simulink library "SCA_SimulinkHIL_lib"  (R2023b)
settings: Solver=VariableStepAuto  StartTime=0.0  StopTime=10.0  RelTol=1e-3
undefined symbols (not defined in the file): a, b, c, DiscIntNeverNeededParam, n
libraries: simulink x11, hdlsllib x8, $bdroot x6, fpga_utils_lib x4
settings Model: Creator=promero  LastModifiedBy=promero

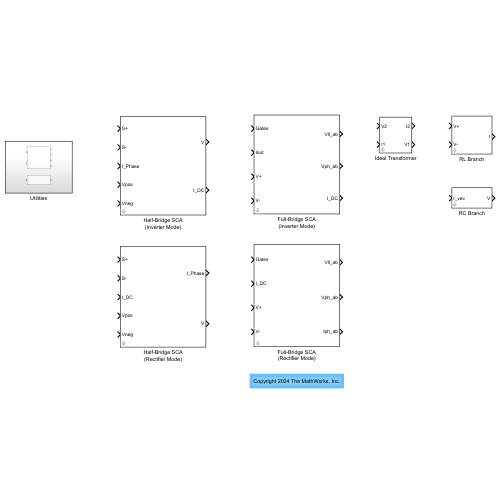
[thumbnail: Simulink's stored preview of the top-level diagram]
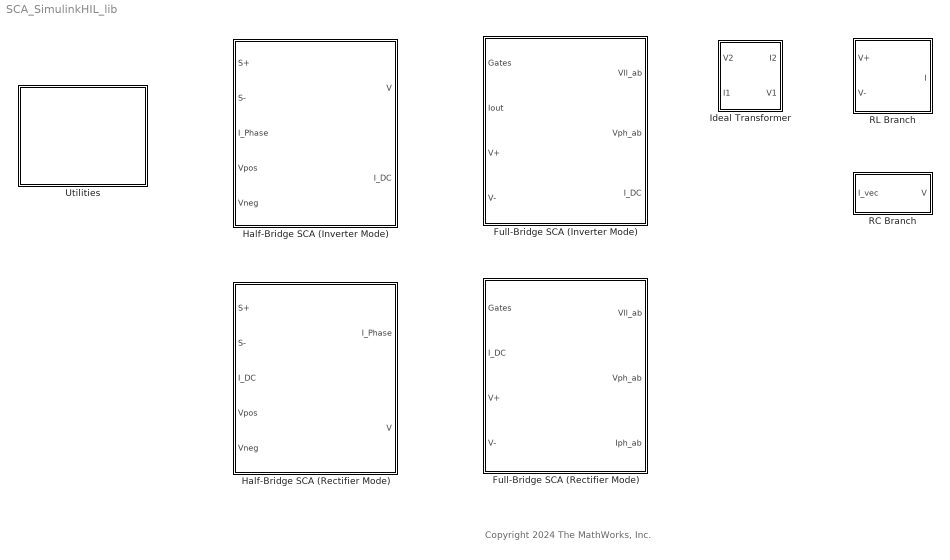
== system SCA_SimulinkHIL_lib ==
  note: Copyright 2024 The MathWorks, Inc.
  Full-Bridge SCA (Inverter Mode) : Subsystem  mask{vfSwitch=0.5, rSwitch=0.001, vfDiode=0.8, rDiode=0.001, avgRatio=1, rSnub=100, useFixedP=on}
      mask prompts: vfSwitch "Switch Threshold [V]"; rSwitch "Switch Closed Resistance [Ohms]"; vfDiode "Diode Forward Voltage [V]"; rDiode "Diode On Resistance [Ohms]"; avgRatio "Subcycle Average Factor [-]"; rSnub "Snubber Resistance [Ohms]"; useFixedP "Use fixed-point implementation"
      mask TypeOptions vfSwitch: Half-Bridge SCA Phase A/vfSwitch | Half-Bridge SCA Phase B/vfSwitch
      mask TypeOptions rSwitch: Half-Bridge SCA Phase A/rSwitch | Half-Bridge SCA Phase B/rSwitch
      mask TypeOptions vfDiode: Half-Bridge SCA Phase A/vfDiode | Half-Bridge SCA Phase B/vfDiode
      mask TypeOptions rDiode: Half-Bridge SCA Phase A/rDiode | Half-Bridge SCA Phase B/rDiode
      mask TypeOptions avgRatio: Half-Bridge SCA Phase A/avgRatio | Half-Bridge SCA Phase B/avgRatio
      mask TypeOptions rSnub: Half-Bridge SCA Phase A/rSnub | Half-Bridge SCA Phase B/rSnub
      mask TypeOptions useFixedP: Half-Bridge SCA Phase A/useFixedP | Half-Bridge SCA Phase B/useFixedP
      mask DialogControl ParameterGroupVar Prompt: Physical Paramaters
      mask DialogControl Container3 Prompt: Simulation Parameters
  Full-Bridge SCA (Rectifier Mode) : Subsystem  mask{vfSwitch=0.5, rSwitch=0.001, cSwitch=1e-8, vfDiode=0.6, rDiode=0.3, cDiode=1e-8, avgRatio=1, rSnubber=1000, useFixedP=on}
      mask prompts: vfSwitch "Switch Threshold [V]"; rSwitch "Switch Closed Resistance [Ohm]"; cSwitch "Switch Open Conductance [1/Ohm]"; vfDiode "Diode Forward Voltage [V]"; rDiode "Diode On Resistance [Ohm]"; cDiode "Diode Off Conductance [1/Ohm]"; avgRatio "Window length"; rSnubber "Snubber Resistance [Ohm]"; useFixedP "Use fixed-point implementation"
      mask TypeOptions vfSwitch:
      | Half-Bridge SCA Phase A
      | (Rectifier Mode)/vfSwitch | Half-Bridge SCA Phase B
      | (Rectifier Mode)/vfSwitch
      mask TypeOptions rSwitch:
      | Half-Bridge SCA Phase A
      | (Rectifier Mode)/rSwitch | Half-Bridge SCA Phase B
      | (Rectifier Mode)/rSwitch
      mask TypeOptions cSwitch:
      | Half-Bridge SCA Phase A
      | (Rectifier Mode)/cSwitch | Half-Bridge SCA Phase B
      | (Rectifier Mode)/cSwitch
      mask TypeOptions vfDiode:
      | Half-Bridge SCA Phase A
      | (Rectifier Mode)/vfDiode | Half-Bridge SCA Phase B
      | (Rectifier Mode)/vfDiode
      mask TypeOptions rDiode:
      | Half-Bridge SCA Phase A
      | (Rectifier Mode)/rDiode | Half-Bridge SCA Phase B
      | (Rectifier Mode)/rDiode
      mask TypeOptions cDiode:
      | Half-Bridge SCA Phase A
      | (Rectifier Mode)/cDiode | Half-Bridge SCA Phase B
      | (Rectifier Mode)/cDiode
      mask TypeOptions avgRatio:
      | Half-Bridge SCA Phase A
      | (Rectifier Mode)/avgRatio | Half-Bridge SCA Phase B
      | (Rectifier Mode)/avgRatio
      mask TypeOptions rSnubber:
      | Half-Bridge SCA Phase A
      | (Rectifier Mode)/rSnubber | Half-Bridge SCA Phase B
      | (Rectifier Mode)/rSnubber
      mask TypeOptions useFixedP:
      | Half-Bridge SCA Phase A
      | (Rectifier Mode)/useFixedP | Half-Bridge SCA Phase B
      | (Rectifier Mode)/useFixedP
      mask DialogControl ParameterGroupVar Prompt: Physical Paramaters
      mask DialogControl Container3 Prompt: Simulation Parameters
  Half-Bridge SCA (Inverter Mode) : Subsystem  mask{vfSwitch=0.5, rSwitch=0.001, vfDiode=0.8, rDiode=0.001, avgRatio=1, useFixedP=on, rSnub=100}
      mask prompts: vfSwitch "Switch Threshold [V]"; rSwitch "Switch Closed Resistance [Ohm]"; vfDiode "Diode Forward Voltage [V]"; rDiode "Diode On Resistance [Ohm]"; avgRatio "Window length"; useFixedP "Use fixed-point implementation"; rSnub "Snubber Resistance [Ohm]"
      mask init:
      | if useFixedP
      |     set_param([gcb,'/Data Type Conversion'],"Commented","through");
      |     set_param([gcb,'/Data Type Conversion1'],"Commented","through");
      |     set_param([gcb,'/Data Type Conversion2'],"Commented","through");
      | else
      |     set_param([gcb,'/Data Type Conversion'],"Commented","off");
      |     set_param([gcb,'/Data Type Conversion1'],"Commented","off");
      |     set_param([gcb,'/Data Type Conversion2'],"Commented","off");
      | end
      mask TypeOptions avgRatio: Switch State Average/avgRatio
      mask DialogControl ParameterGroupVar Prompt: Physical Parameters
      mask DialogControl Container3 Prompt: Simulation Parameters
  Half-Bridge SCA (Rectifier Mode) : Subsystem  mask{vfSwitch=0.5, rSwitch=0.001, cSwitch=1e-8, vfDiode=0.6, rDiode=0.3, cDiode=1e-8, avgRatio=1, useFixedP=on, rSnubber=inf}
      mask prompts: vfSwitch "Switch Threshold [V]"; rSwitch "Switch Closed Resistance [Ohm]"; cSwitch "Switch Open Conductance [1/Ohm]"; vfDiode "Diode Forward Voltage [V]"; rDiode "Diode On Resistance [Ohm]"; cDiode "Diode Off Conductance [1/Ohm]"; avgRatio "Window length"; useFixedP "Use fixed-point implementation"; rSnubber "Snubber Resistance [Ohm]"
      mask init:
      | if rDiode > 0
      |     rEquiv = 1/(1/rSwitch + 1/rDiode);
      | else
      |     rEquiv = rSwitch;
      | end
      | 
      | if useFixedP
      |     set_param([gcb,'/Data Type Conversion'],"Commented","through");
      |     set_param([gcb,'/Data Type Conversion1'],"Commented","through");
      |     set_param([gcb,'/Data Type Conversion2'],"Commented","through");
      | else
      |     set_param([gcb,'/Data Type Conversion'],"Commented","off");
      |     set_param([gcb,'/Data Type Conversion1'],"Commented","off");
      |     set_param([gcb,'/Data Type Conversion2'],"Commented","off");
      | end
      mask TypeOptions avgRatio: Switch State Average/avgRatio
      mask DialogControl ParameterGroupVar Prompt: Physical Parameters
      mask DialogControl Container3 Prompt: Simulation Parameters
  Ideal Transformer : Subsystem  mask(Ideal Transformer){Parameter1=1}
      mask prompts: Parameter1 "Winding ratio [-]"
  RC Branch : Subsystem  mask(RC Branch){C=1e-4, R=0.1}
      mask prompts: C "Capacitance [F]"; R "Resistance [Ohm]"
  RL Branch : Subsystem  mask(RL Branch){L=1e-6, R=0}
      mask prompts: L "Inductance [H]"; R "Resistance [Ohm]"
  Utilities : Subsystem

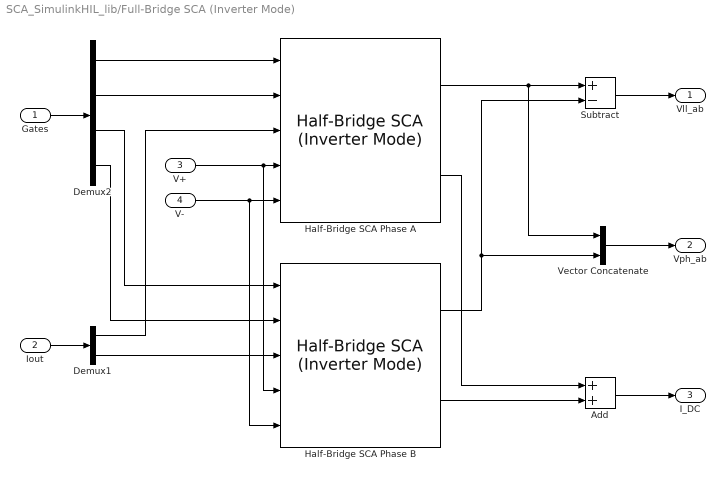
== system SCA_SimulinkHIL_lib/Full-Bridge SCA (Inverter Mode) ==
  Gates : Inport  OutDataTypeStr=boolean  PortDimensions=4
  Iout : Inport  Port=2  PortDimensions=2
  V+ : Inport  Port=3  PortDimensions=1
  V- : Inport  Port=4  PortDimensions=1
  Add : Sum
  Demux1 : Demux  Outputs=2
  Demux2 : Demux
  Half-Bridge SCA Phase A : $bdroot/Half-Bridge SCA (Inverter Mode)  vfSwitch=vfSwitch  rSwitch=rSwitch  vfDiode=vfDiode  rDiode=rDiode  avgRatio=avgRatio  useFixedP=on  rSnub=rSnub
  Half-Bridge SCA Phase B : $bdroot/Half-Bridge SCA (Inverter Mode)  vfSwitch=vfSwitch  rSwitch=rSwitch  vfDiode=vfDiode  rDiode=rDiode  avgRatio=avgRatio  useFixedP=on  rSnub=rSnub
  Subtract : Sum  Inputs=+-
  Vector Concatenate : Concatenate
  Vll_ab : Outport
  Vph_ab : Outport  Port=2
  I_DC : Outport  Port=3
  wires:
  Demux2/2 -> Half-Bridge SCA Phase A/2
  Demux2/1 -> Half-Bridge SCA Phase A/1
  Gates/1 -> Demux2/1
  Demux2/3 -> Half-Bridge SCA Phase B/1
  Demux2/4 -> Half-Bridge SCA Phase B/2
  Iout/1 -> Demux1/1
  Demux1/1 -> Half-Bridge SCA Phase A/3
  Demux1/2 -> Half-Bridge SCA Phase B/3
  V+/1 -> Half-Bridge SCA Phase B/4, Half-Bridge SCA Phase A/4
  V-/1 -> Half-Bridge SCA Phase B/5, Half-Bridge SCA Phase A/5
  Half-Bridge SCA Phase A/2 -> Add/1
  Half-Bridge SCA Phase B/2 -> Add/2
  Add/1 -> I_DC/1
  Half-Bridge SCA Phase A/1 -> Vector Concatenate/1, Subtract/1
  Half-Bridge SCA Phase B/1 -> Vector Concatenate/2, Subtract/2
  Subtract/1 -> Vll_ab/1
  Vector Concatenate/1 -> Vph_ab/1

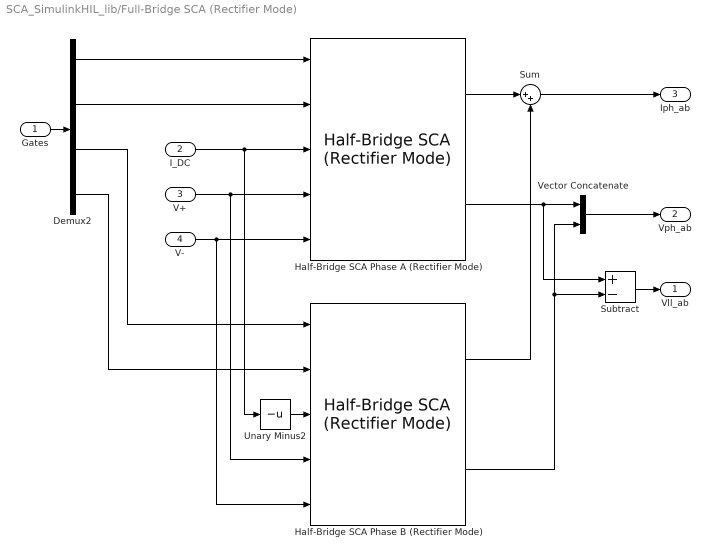
== system SCA_SimulinkHIL_lib/Full-Bridge SCA (Rectifier Mode) ==
  Gates : Inport  PortDimensions=4
  I_DC : Inport  Port=2  PortDimensions=1
  V+ : Inport  Port=3  PortDimensions=1
  V- : Inport  Port=4  PortDimensions=1
  Demux2 : Demux
  Half-Bridge SCA Phase A (Rectifier Mode) : $bdroot/Half-Bridge SCA (Rectifier Mode)  vfSwitch=vfSwitch  rSwitch=rSwitch  cSwitch=cSwitch  vfDiode=vfDiode  rDiode=rDiode  cDiode=cDiode  avgRatio=avgRatio  useFixedP=on  rSnubber=rSnubber
  Half-Bridge SCA Phase B (Rectifier Mode) : $bdroot/Half-Bridge SCA (Rectifier Mode)  vfSwitch=vfSwitch  rSwitch=rSwitch  cSwitch=cSwitch  vfDiode=vfDiode  rDiode=rDiode  cDiode=cDiode  avgRatio=avgRatio  useFixedP=on  rSnubber=rSnubber
  Subtract : Sum  Inputs=+-  OutDataTypeStr=Inherit: Inherit via back propagation
  Sum : Sum  Inputs=|++
  Unary Minus2 : UnaryMinus
  Vector Concatenate : Concatenate
  Vll_ab : Outport
  Vph_ab : Outport  Port=2
  Iph_ab : Outport  Port=3
  wires:
  V-/1 -> Half-Bridge SCA Phase A (Rectifier Mode)/5, Half-Bridge SCA Phase B (Rectifier Mode)/5
  V+/1 -> Half-Bridge SCA Phase A (Rectifier Mode)/4, Half-Bridge SCA Phase B (Rectifier Mode)/4
  I_DC/1 -> Half-Bridge SCA Phase A (Rectifier Mode)/3, Unary Minus2/1
  Unary Minus2/1 -> Half-Bridge SCA Phase B (Rectifier Mode)/3
  Half-Bridge SCA Phase B (Rectifier Mode)/2 -> Subtract/2, Vector Concatenate/2
  Vector Concatenate/1 -> Vph_ab/1
  Sum/1 -> Iph_ab/1
  Half-Bridge SCA Phase A (Rectifier Mode)/2 -> Subtract/1, Vector Concatenate/1
  Half-Bridge SCA Phase B (Rectifier Mode)/1 -> Sum/2
  Half-Bridge SCA Phase A (Rectifier Mode)/1 -> Sum/1
  Demux2/4 -> Half-Bridge SCA Phase B (Rectifier Mode)/2
  Gates/1 -> Demux2/1
  Demux2/2 -> Half-Bridge SCA Phase A (Rectifier Mode)/2
  Demux2/1 -> Half-Bridge SCA Phase A (Rectifier Mode)/1
  Demux2/3 -> Half-Bridge SCA Phase B (Rectifier Mode)/1
  Subtract/1 -> Vll_ab/1

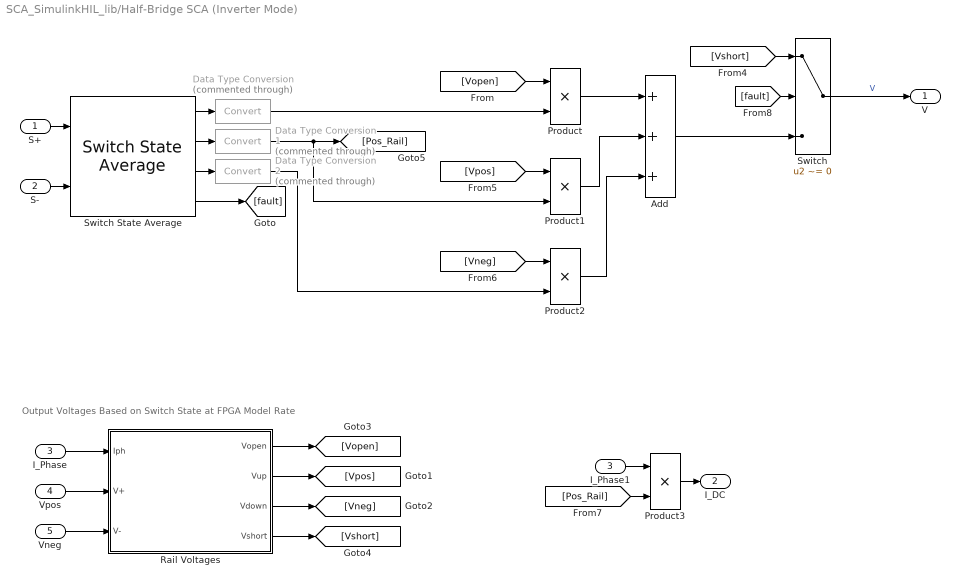
== system SCA_SimulinkHIL_lib/Half-Bridge SCA (Inverter Mode) ==
  note: Output Voltages Based on Switch State at FPGA Model Rate
  S+ : Inport
  S- : Inport  Port=2
  I_Phase : Inport  Port=3
  Vpos : Inport  Port=4
  Vneg : Inport  Port=5
  Add : Sum  Inputs=+++  OutDataTypeStr=Inherit: Inherit via back propagation
  Data Type Conversion : DataTypeConversion  Commented=through  SaturateOnIntegerOverflow=off  RndMeth=Floor
  Data Type Conversion1 : DataTypeConversion  Commented=through  SaturateOnIntegerOverflow=off  RndMeth=Floor
  Data Type Conversion2 : DataTypeConversion  Commented=through  SaturateOnIntegerOverflow=off  RndMeth=Floor
  I_Phase1 : InportShadow  Port=3
  Product{,1..3} (4 alike) : Product  OutDataTypeStr=Inherit: Same as first input
  Rail Voltages : Subsystem
  Switch : Switch  Criteria=u2 ~= 0  SaturateOnIntegerOverflow=off
  Switch State Average : $bdroot/Utilities/Switch State Average  avgRatio=avgRatio
  V : Outport  VectorParamsAs1DForOutWhenUnconnected=off
  I_DC : Outport  Port=2  VectorParamsAs1DForOutWhenUnconnected=off
  wires:
  [Vshort] -> Switch/1
  Switch/1 -> V/1  "V"
  [fault] -> Switch/2
  Switch State Average/2 -> Data Type Conversion1/1
  [Vpos] -> Product1/1
  [Pos_Rail] -> Product3/2
  I_Phase1/1 -> Product3/1
  Vpos/1 -> Rail Voltages/2(V+)
  Vneg/1 -> Rail Voltages/3(V-)
  Rail Voltages/1(Vopen) -> [Vopen]
  Rail Voltages/2(Vup) -> [Vpos]
  Rail Voltages/3(Vdown) -> [Vneg]
  Rail Voltages/4(Vshort) -> [Vshort]
  Switch State Average/4 -> [fault]
  S+/1 -> Switch State Average/1
  S-/1 -> Switch State Average/2
  Add/1 -> Switch/3
  I_Phase/1 -> Rail Voltages/1(Iph)
  [Vopen] -> Product/1
  Switch State Average/1 -> Data Type Conversion/1
  Product/1 -> Add/1
  [Vneg] -> Product2/1
  Switch State Average/3 -> Data Type Conversion2/1
  Product1/1 -> Add/2
  Product2/1 -> Add/3
  Product3/1 -> I_DC/1
  Data Type Conversion/1 -> Product/2
  Data Type Conversion1/1 -> Product1/2, [Pos_Rail]
  Data Type Conversion2/1 -> Product2/2

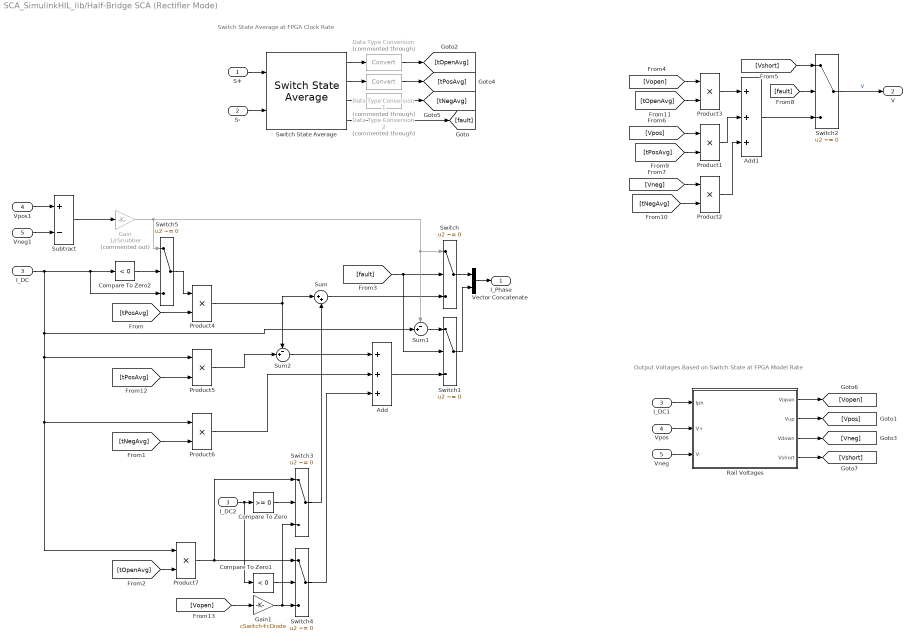
== system SCA_SimulinkHIL_lib/Half-Bridge SCA (Rectifier Mode) ==
  note: Switch State Average at FPGA Clock Rate
  note: Output Voltages Based on Switch State at FPGA Model Rate
  S+ : Inport  PortDimensions=1
  S- : Inport  Port=2  PortDimensions=1
  I_DC : Inport  Port=3
  Vpos : Inport  Port=4
  Vneg : Inport  Port=5
  Add : Sum  Inputs=+++  OutDataTypeStr=Inherit: Inherit via back propagation
  Add1 : Sum  Inputs=+++  OutDataTypeStr=Inherit: Inherit via back propagation  InputSameDT=on
  Compare To Zero : simulink/Logic and Bit Operations/Compare To Zero  relop=>=  OutDataTypeStr=boolean
  Compare To Zero1 : simulink/Logic and Bit Operations/Compare To Zero  relop=<  OutDataTypeStr=boolean
  Compare To Zero2 : simulink/Logic and Bit Operations/Compare To Zero  relop=<  OutDataTypeStr=boolean
  Data Type Conversion : DataTypeConversion  Commented=through  SaturateOnIntegerOverflow=off  RndMeth=Floor
  Data Type Conversion1 : DataTypeConversion  Commented=through  SaturateOnIntegerOverflow=off  RndMeth=Floor
  Data Type Conversion2 : DataTypeConversion  Commented=through  SaturateOnIntegerOverflow=off  RndMeth=Floor
  Gain : Gain  Commented=on  Gain=1/rSnubber  OutDataTypeStr=Inherit: Inherit via back propagation
  Gain1 : Gain  Gain=cSwitch+cDiode  OutDataTypeStr=Inherit: Inherit via back propagation
  I_DC1 : InportShadow  Port=3
  I_DC2 : InportShadow  Port=3
  Product{1..7} (7 alike) : Product  OutDataTypeStr=Inherit: Same as first input
  Rail Voltages : Subsystem
  Subtract : Sum  Inputs=+-
  Sum : Sum  Inputs=|++  OutDataTypeStr=Inherit: Inherit via back propagation
  Sum1 : Sum  Inputs=-+|  OutDataTypeStr=Inherit: Inherit via back propagation
  Sum2 : Sum  Inputs=-+|
  Switch{,1..5} (6 alike) : Switch  Criteria=u2 ~= 0  SaturateOnIntegerOverflow=off
  Switch State Average : $bdroot/Utilities/Switch State Average  avgRatio=avgRatio
  Vector Concatenate : Concatenate
  Vneg1 : InportShadow  Port=5
  Vpos1 : InportShadow  Port=4
  I_Phase : Outport
  V : Outport  Port=2  VectorParamsAs1DForOutWhenUnconnected=off
  wires:
  Sum2/1 -> Add/1
  Switch4/1 -> Add/3
  Add/1 -> Switch1/3
  Switch5/1 -> Product4/1
  Compare To Zero2/1 -> Switch5/2
  Compare To Zero1/1 -> Switch4/2
  Switch3/1 -> Sum/2
  Product7/1 -> Switch3/1, Switch4/1
  Compare To Zero/1 -> Switch3/2
  I_DC2/1 -> Compare To Zero/1, Compare To Zero1/1
  Vneg1/1 -> Subtract/2
  Vpos1/1 -> Subtract/1
  Sum1/1 -> Switch1/1
  [fault] -> Switch1/2, Switch/2
  Sum/1 -> Switch/3
  I_DC/1 -> Compare To Zero2/1, Switch5/3, Product5/1, Product7/1, Product6/1, Sum1/2
  [tPosAvg] -> Product4/2
  Switch State Average/1 -> Data Type Conversion/1
  Switch State Average/2 -> Data Type Conversion1/1
  Switch State Average/3 -> Data Type Conversion2/1
  Switch State Average/4 -> [fault]
  Rail Voltages/4(Vshort) -> [Vshort]
  Vneg/1 -> Rail Voltages/3(V-)
  Vpos/1 -> Rail Voltages/2(V+)
  Rail Voltages/1(Vopen) -> [Vopen]
  Rail Voltages/2(Vup) -> [Vpos]
  I_DC1/1 -> Rail Voltages/1(Iph)
  Rail Voltages/3(Vdown) -> [Vneg]
  [Vopen] -> Product3/1
  Switch2/1 -> V/1  "V"
  Add1/1 -> Switch2/3
  [Vshort] -> Switch2/1
  [Vneg] -> Product2/1
  [fault] -> Switch2/2
  [tOpenAvg] -> Product3/2
  [tNegAvg] -> Product2/2
  Vector Concatenate/1 -> I_Phase/1
  Switch/1 -> Vector Concatenate/1
  Switch1/1 -> Vector Concatenate/2
  S+/1 -> Switch State Average/1
  S-/1 -> Switch State Average/2
  Subtract/1 -> Gain/1
  Gain/1 -> Switch/1, Sum1/1, Switch5/1
  [Vopen] -> Gain1/1
  Gain1/1 -> Switch4/3, Switch3/3
  [Vpos] -> Product1/1
  [tPosAvg] -> Product1/2
  Product3/1 -> Add1/1
  Product1/1 -> Add1/2
  Product2/1 -> Add1/3
  Product4/1 -> Sum/1, Sum2/1
  Product5/1 -> Sum2/2
  [tPosAvg] -> Product5/2
  [tNegAvg] -> Product6/2
  Product6/1 -> Add/2
  [tOpenAvg] -> Product7/2
  Data Type Conversion/1 -> [tOpenAvg]
  Data Type Conversion1/1 -> [tPosAvg]
  Data Type Conversion2/1 -> [tNegAvg]

== system SCA_SimulinkHIL_lib/Ideal Transformer ==
  V2 : Inport  PortDimensions=1
  I1 : Inport  Port=2
  Gain1 : Gain  Gain=n  OutDataTypeStr=Inherit: Inherit via back propagation
  Gain2 : Gain  Gain=n  OutDataTypeStr=Inherit: Inherit via back propagation
  I2 : Outport
  V1 : Outport  Port=2
  wires:
  V2/1 -> Gain2/1
  Gain2/1 -> V1/1
  Gain1/1 -> I2/1
  I1/1 -> Gain1/1

== system SCA_SimulinkHIL_lib/RC Branch ==
  I_vec : Inport
  Constant : Constant  Value=R  OutDataTypeStr=Inherit: Inherit via back propagation  SampleTime=Inf
  Data Type Duplicate : DataTypeDuplicate
  Discrete-Time Integrator : DiscreteIntegrator  gainval=1/C  SampleTime=-1  OutDataTypeStr=Inherit: Inherit via back propagation  ICPrevOutput=DiscIntNeverNeededParam  ICPrevScaledInput=DiscIntNeverNeededParam
  Multiply-Add : hdlsllib/HDL Operations/Multiply-Add  Function=c-(a.*b)  datatype=Inherit: Inherit via back propagation  DoSatur=off  FMA=off
  Sum of Elements : Sum  Inputs=+
  V : Outport
  wires:
  Sum of Elements/1 -> Multiply-Add/1, Discrete-Time Integrator/1
  I_vec/1 -> Sum of Elements/1
  Constant/1 -> Multiply-Add/2
  Discrete-Time Integrator/1 -> Data Type Duplicate/2, Multiply-Add/3
  Multiply-Add/1 -> Data Type Duplicate/1, V/1

== system SCA_SimulinkHIL_lib/RL Branch ==
  V+ : Inport  PortDimensions=1
  V- : Inport  Port=2  PortDimensions=1
  Discrete-Time Integrator : DiscreteIntegrator  gainval=1/L  SampleTime=-1  OutDataTypeStr=Inherit: Inherit via back propagation  ICPrevOutput=DiscIntNeverNeededParam  ICPrevScaledInput=DiscIntNeverNeededParam
  Gain : Gain  Gain=R  OutDataTypeStr=Inherit: Inherit via back propagation
  Subtract : Sum  Inputs=+--  OutDataTypeStr=Inherit: Inherit via back propagation
  Unit Delay : UnitDelay  SampleTime=-1  HasFrameUpgradeWarning=on
  I : Outport
  wires:
  Discrete-Time Integrator/1 -> Gain/1, I/1
  V+/1 -> Subtract/1
  Subtract/1 -> Discrete-Time Integrator/1
  V-/1 -> Subtract/2
  Gain/1 -> Unit Delay/1
  Unit Delay/1 -> Subtract/3

== system SCA_SimulinkHIL_lib/Utilities ==
  Fast to Slow Transition : Subsystem  mask{avgRatio=1}
      mask prompts: avgRatio "Time scaling factor"
      mask TypeOptions avgRatio: HDL Moving Average/avgRatio | Rate Transition/OutPortSampleTimeMultiple
  Switch State Average : Subsystem  mask{avgRatio=1}
      mask prompts: avgRatio "Window length"
      mask TypeOptions avgRatio: Subsystem/Moving Average/HDL Moving Average/avgRatio | Subsystem/Moving Average/HDL Moving Average1/avgRatio | Subsystem/Moving Average/HDL Moving Average2/avgRatio
      mask DialogControl Container3 Prompt: Parameters

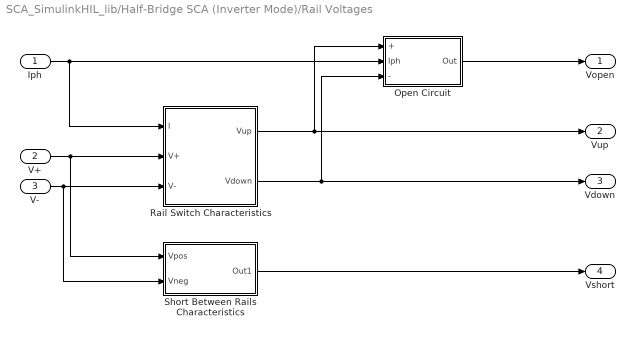
== system SCA_SimulinkHIL_lib/Half-Bridge SCA (Inverter Mode)/Rail Voltages ==
  Iph : Inport
  V+ : Inport  Port=2
  V- : Inport  Port=3
  Open Circuit : Subsystem
  Rail Switch Characteristics : Subsystem
  Short Between Rails Characteristics : Subsystem
  Vopen : Outport
  Vup : Outport  Port=2
  Vdown : Outport  Port=3
  Vshort : Outport  Port=4
  wires:
  Open Circuit/1(Out) -> Vopen/1
  V-/1 -> Short Between Rails Characteristics/2(Vneg), Rail Switch Characteristics/3(V-)
  Rail Switch Characteristics/2(Vdown) -> Open Circuit/3(-), Vdown/1
  Rail Switch Characteristics/1(Vup) -> Open Circuit/1(+), Vup/1
  V+/1 -> Rail Switch Characteristics/2(V+), Short Between Rails Characteristics/1(Vpos)
  Short Between Rails Characteristics/1(Out1) -> Vshort/1
  Iph/1 -> Rail Switch Characteristics/1(I), Open Circuit/2(Iph)

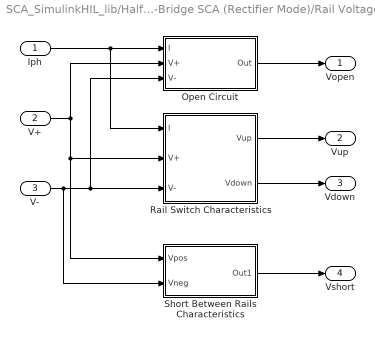
== system SCA_SimulinkHIL_lib/Half-Bridge SCA (Rectifier Mode)/Rail Voltages ==
  Iph : Inport
  V+ : Inport  Port=2
  V- : Inport  Port=3
  Open Circuit : Subsystem
  Rail Switch Characteristics : Subsystem
  Short Between Rails Characteristics : Subsystem
  Vopen : Outport
  Vup : Outport  Port=2
  Vdown : Outport  Port=3
  Vshort : Outport  Port=4
  wires:
  Open Circuit/1(Out) -> Vopen/1
  V-/1 -> Open Circuit/3(V-), Rail Switch Characteristics/3(V-), Short Between Rails Characteristics/2(Vneg)
  Iph/1 -> Rail Switch Characteristics/1(I), Open Circuit/1(I)
  Rail Switch Characteristics/1(Vup) -> Vup/1
  V+/1 -> Short Between Rails Characteristics/1(Vpos), Rail Switch Characteristics/2(V+), Open Circuit/2(V+)
  Short Between Rails Characteristics/1(Out1) -> Vshort/1
  Rail Switch Characteristics/2(Vdown) -> Vdown/1

== system SCA_SimulinkHIL_lib/Utilities/Fast to Slow Transition ==
  In : Inport
  Data Type Duplicate1 : DataTypeDuplicate
  HDL Moving Average : fpga_utils_lib/HDL Moving Average  avgRatio=avgRatio
  Rate Transition : RateTransition  OutPortSampleTimeOpt=Multiple of input port sample time  OutPortSampleTimeMultiple=avgRatio
  Out : Outport
  wires:
  HDL Moving Average/1 -> Data Type Duplicate1/1, Rate Transition/1
  In/1 -> Data Type Duplicate1/2, HDL Moving Average/1
  Rate Transition/1 -> Out/1

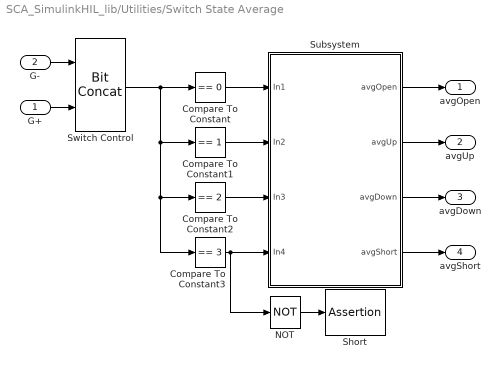
== system SCA_SimulinkHIL_lib/Utilities/Switch State Average ==
  G+ : Inport  OutDataTypeStr=boolean  PortDimensions=1
  G- : Inport  Port=2  OutDataTypeStr=boolean  PortDimensions=1
  Compare To Constant : simulink/Logic and Bit Operations/Compare To Constant  relop===  const=0  OutDataTypeStr=boolean
  Compare To Constant1 : simulink/Logic and Bit Operations/Compare To Constant  relop===  const=1  OutDataTypeStr=boolean
  Compare To Constant2 : simulink/Logic and Bit Operations/Compare To Constant  relop===  const=2  OutDataTypeStr=boolean
  Compare To Constant3 : simulink/Logic and Bit Operations/Compare To Constant  relop===  const=3  OutDataTypeStr=boolean
  NOT : Logic  Operator=NOT  IconShape=distinctive  AllPortsSameDT=off  OutDataTypeStr=boolean
  Short : Assertion  StopWhenAssertionFail=off
  Subsystem : Subsystem  Variant=on  VariantControl=Subsystem
  Switch Control : hdlsllib/Logic and Bit Operations/Bit Concat  numInputs=2
  avgOpen : Outport
  avgUp : Outport  Port=2
  avgDown : Outport  Port=3
  avgShort : Outport  Port=4
  wires:
  Switch Control/1 -> Compare To Constant/1, Compare To Constant3/1, Compare To Constant2/1, Compare To Constant1/1
  NOT/1 -> Short/1
  Compare To Constant3/1 -> NOT/1, Subsystem/4(In4)
  G+/1 -> Switch Control/2
  G-/1 -> Switch Control/1
  Compare To Constant/1 -> Subsystem/1(In1)
  Compare To Constant1/1 -> Subsystem/2(In2)
  Compare To Constant2/1 -> Subsystem/3(In3)
  Subsystem/1(avgOpen) -> avgOpen/1
  Subsystem/2(avgUp) -> avgUp/1
  Subsystem/3(avgDown) -> avgDown/1
  Subsystem/4(avgShort) -> avgShort/1

== system SCA_SimulinkHIL_lib/Half-Bridge SCA (Inverter Mode)/Rail Voltages/Open Circuit ==
  + : Inport
  Iph : Inport  Port=2
  - : Inport  Port=3
  Gain : Gain  Gain=-rSnub
  Saturation Dynamic : simulink/Discontinuities/Saturation Dynamic  OutMin=[]  OutMax=[]  OutDataTypeStr=Inherit: Inherit via back propagation  OutDataType=fixdt(1, 16)  OutScaling=2^-10  DoSatur=off
  Out : Outport  VectorParamsAs1DForOutWhenUnconnected=off
  wires:
  Iph/1 -> Gain/1
  Gain/1 -> Saturation Dynamic/2
  Saturation Dynamic/1 -> Out/1
  +/1 -> Saturation Dynamic/1
  -/1 -> Saturation Dynamic/3

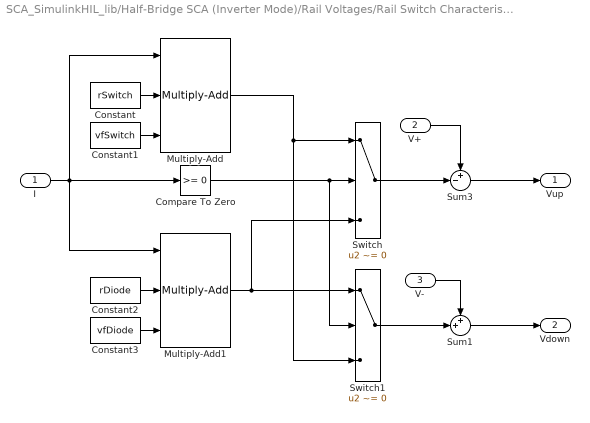
== system SCA_SimulinkHIL_lib/Half-Bridge SCA (Inverter Mode)/Rail Voltages/Rail Switch Characteristics ==
  I : Inport
  V+ : Inport  Port=2
  V- : Inport  Port=3
  Compare To Zero : simulink/Logic and Bit Operations/Compare To Zero  relop=>=  OutDataTypeStr=boolean
  Constant : Constant  Value=rSwitch  OutDataTypeStr=Inherit: Inherit via back propagation
  Constant1 : Constant  Value=vfSwitch  OutDataTypeStr=Inherit: Inherit via back propagation
  Constant2 : Constant  Value=rDiode  OutDataTypeStr=Inherit: Inherit via back propagation
  Constant3 : Constant  Value=vfDiode  OutDataTypeStr=Inherit: Inherit via back propagation
  Multiply-Add : hdlsllib/HDL Operations/Multiply-Add  Function=c+(a.*b)  datatype=Inherit: Inherit via back propagation  DoSatur=off  FMA=off
  Multiply-Add1 : hdlsllib/HDL Operations/Multiply-Add  Function=(a.*b)-c  datatype=Inherit: Inherit via back propagation  DoSatur=off  FMA=off
  Sum1 : Sum  Inputs=++|  OutDataTypeStr=Inherit: Same as first input
  Sum3 : Sum  Inputs=+-|  OutDataTypeStr=Inherit: Same as first input
  Switch : Switch  Criteria=u2 ~= 0  SaturateOnIntegerOverflow=off  InputSameDT=off
  Switch1 : Switch  Criteria=u2 ~= 0  SaturateOnIntegerOverflow=off  InputSameDT=off
  Vup : Outport  VectorParamsAs1DForOutWhenUnconnected=off
  Vdown : Outport  Port=2  VectorParamsAs1DForOutWhenUnconnected=off
  wires:
  Switch/1 -> Sum3/2
  V+/1 -> Sum3/1
  Sum3/1 -> Vup/1
  I/1 -> Compare To Zero/1, Multiply-Add/1, Multiply-Add1/1
  Switch1/1 -> Sum1/2
  Sum1/1 -> Vdown/1
  V-/1 -> Sum1/1
  Compare To Zero/1 -> Switch1/2, Switch/2
  Multiply-Add/1 -> Switch1/3, Switch/1
  Constant/1 -> Multiply-Add/2
  Constant1/1 -> Multiply-Add/3
  Multiply-Add1/1 -> Switch/3, Switch1/1
  Constant2/1 -> Multiply-Add1/2
  Constant3/1 -> Multiply-Add1/3

== system SCA_SimulinkHIL_lib/Half-Bridge SCA (Inverter Mode)/Rail Voltages/Short Between Rails Characteristics ==
  Vpos : Inport
  Vneg : Inport  Port=2
  Gain : Gain  Gain=1/2  OutDataTypeStr=Inherit: Inherit via back propagation
  Subtract : Sum  Inputs=+-
  Out1 : Outport
  wires:
  Vpos/1 -> Subtract/1
  Gain/1 -> Out1/1
  Vneg/1 -> Subtract/2
  Subtract/1 -> Gain/1

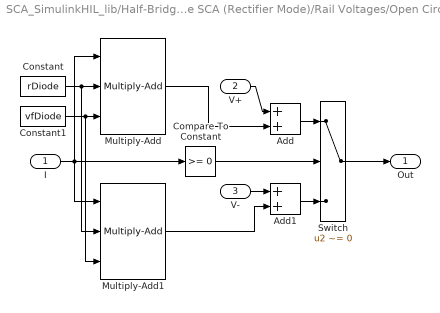
== system SCA_SimulinkHIL_lib/Half-Bridge SCA (Rectifier Mode)/Rail Voltages/Open Circuit ==
  I : Inport
  V+ : Inport  Port=2
  V- : Inport  Port=3
  Add : Sum  OutDataTypeStr=Inherit: Same as first input
  Add1 : Sum  OutDataTypeStr=Inherit: Same as first input
  Compare To Constant : simulink/Logic and Bit Operations/Compare To Constant  relop=>=  const=0  OutDataTypeStr=boolean
  Constant : Constant  Value=rDiode  OutDataTypeStr=Inherit: Inherit via back propagation
  Constant1 : Constant  Value=vfDiode  OutDataTypeStr=Inherit: Inherit via back propagation
  Multiply-Add : hdlsllib/HDL Operations/Multiply-Add  Function=c+(a.*b)  datatype=Inherit: Inherit via internal rule  DoSatur=off  FMA=off
  Multiply-Add1 : hdlsllib/HDL Operations/Multiply-Add  Function=(a.*b)-c  datatype=Inherit: Inherit via internal rule  DoSatur=off  FMA=off
  Switch : Switch  Criteria=u2 ~= 0  SaturateOnIntegerOverflow=off
  Out : Outport  VectorParamsAs1DForOutWhenUnconnected=off
  wires:
  Compare To Constant/1 -> Switch/2
  Switch/1 -> Out/1
  I/1 -> Multiply-Add1/1, Multiply-Add/1, Compare To Constant/1
  Add/1 -> Switch/1
  Multiply-Add/1 -> Add/2
  V+/1 -> Add/1
  Add1/1 -> Switch/3
  Constant/1 -> Multiply-Add1/2, Multiply-Add/2
  Constant1/1 -> Multiply-Add1/3, Multiply-Add/3
  V-/1 -> Add1/1
  Multiply-Add1/1 -> Add1/2

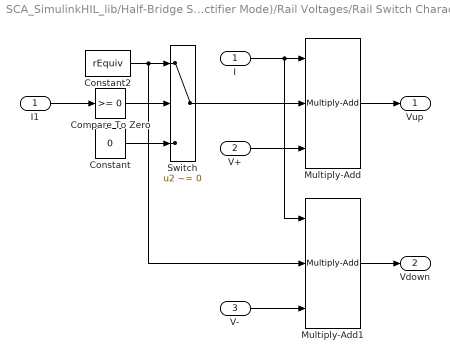
== system SCA_SimulinkHIL_lib/Half-Bridge SCA (Rectifier Mode)/Rail Voltages/Rail Switch Characteristics ==
  I : Inport
  V+ : Inport  Port=2
  V- : Inport  Port=3
  Compare To Zero : simulink/Logic and Bit Operations/Compare To Zero  relop=>=  OutDataTypeStr=boolean
  Constant : Constant  Value=0  OutDataTypeStr=Inherit: Inherit via back propagation  SampleTime=Inf
  Constant2 : Constant  Value=rEquiv  OutMin=0  OutMax=1  OutDataTypeStr=fixdt(1,16)  SampleTime=Inf
  I1 : InportShadow
  Multiply-Add : hdlsllib/HDL Operations/Multiply-Add  Function=c+(a.*b)  datatype=Inherit: Inherit via back propagation  DoSatur=off  FMA=off
  Multiply-Add1 : hdlsllib/HDL Operations/Multiply-Add  Function=c+(a.*b)  datatype=Inherit: Inherit via back propagation  DoSatur=off  FMA=off
  Switch : Switch  Criteria=u2 ~= 0  OutDataTypeStr=Inherit: Inherit via back propagation  SaturateOnIntegerOverflow=off
  Vup : Outport  VectorParamsAs1DForOutWhenUnconnected=off
  Vdown : Outport  Port=2  VectorParamsAs1DForOutWhenUnconnected=off
  wires:
  Constant/1 -> Switch/3
  Compare To Zero/1 -> Switch/2
  Multiply-Add/1 -> Vup/1
  Multiply-Add1/1 -> Vdown/1
  I/1 -> Multiply-Add1/1, Multiply-Add/1
  V+/1 -> Multiply-Add/3
  V-/1 -> Multiply-Add1/3
  Constant2/1 -> Multiply-Add1/2, Switch/1
  Switch/1 -> Multiply-Add/2
  I1/1 -> Compare To Zero/1

== system SCA_SimulinkHIL_lib/Half-Bridge SCA (Rectifier Mode)/Rail Voltages/Short Between Rails Characteristics ==
  Vpos : Inport
  Vneg : Inport  Port=2
  Subtract : Sum  Inputs=+-  OutDataTypeStr=Inherit: Inherit via back propagation
  Out1 : Outport
  wires:
  Vpos/1 -> Subtract/1
  Subtract/1 -> Out1/1
  Vneg/1 -> Subtract/2

== system SCA_SimulinkHIL_lib/Utilities/Switch State Average/Subsystem ==
  In1 : Inport
  In2 : Inport  Port=2
  In3 : Inport  Port=3
  In4 : Inport  Port=4
  Bypass : Subsystem  VariantControl=avgRatio==1
  Moving Average : Subsystem  VariantControl=avgRatio>1
  avgOpen : Outport
  avgUp : Outport  Port=2
  avgDown : Outport  Port=3
  avgShort : Outport  Port=4

== system SCA_SimulinkHIL_lib/Utilities/Switch State Average/Subsystem/Bypass ==
  In1 : Inport
  In2 : Inport  Port=2
  In3 : Inport  Port=3
  In4 : Inport  Port=4
  avgOpen : Outport
  avgUp : Outport  Port=2
  avgDown : Outport  Port=3
  avgShort : Outport  Port=4
  wires:
  In1/1 -> avgOpen/1
  In2/1 -> avgUp/1
  In3/1 -> avgDown/1
  In4/1 -> avgShort/1

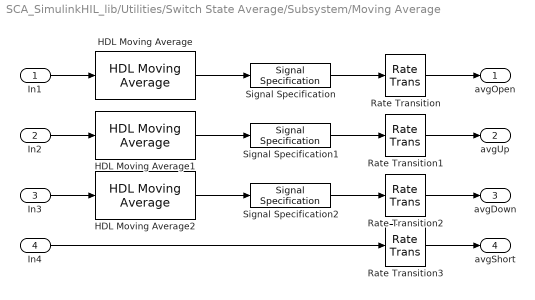
== system SCA_SimulinkHIL_lib/Utilities/Switch State Average/Subsystem/Moving Average ==
  In1 : Inport
  In2 : Inport  Port=2
  In3 : Inport  Port=3
  In4 : Inport  Port=4
  HDL Moving Average : fpga_utils_lib/HDL Moving Average  avgRatio=avgRatio
  HDL Moving Average1 : fpga_utils_lib/HDL Moving Average  avgRatio=avgRatio
  HDL Moving Average2 : fpga_utils_lib/HDL Moving Average  avgRatio=avgRatio
  Rate Transition{,1..3} (4 alike) : RateTransition  OutPortSampleTimeOpt=Multiple of input port sample time  OutPortSampleTimeMultiple=avgRatio
  Signal Specification : SignalSpecification  OutMin=0  OutMax=1  OutDataTypeStr=fixdt(1,15,13)
      settings: LockScale=on
  Signal Specification1 : SignalSpecification  OutMin=0  OutMax=1  OutDataTypeStr=fixdt(1,15,13)
      settings: LockScale=on
  Signal Specification2 : SignalSpecification  OutMin=0  OutMax=1  OutDataTypeStr=fixdt(1,15,13)
      settings: LockScale=on
  avgOpen : Outport
  avgUp : Outport  Port=2
  avgDown : Outport  Port=3
  avgShort : Outport  Port=4
  wires:
  In3/1 -> HDL Moving Average2/1
  Signal Specification/1 -> Rate Transition/1
  Signal Specification2/1 -> Rate Transition2/1
  HDL Moving Average1/1 -> Signal Specification1/1
  HDL Moving Average/1 -> Signal Specification/1
  In4/1 -> Rate Transition3/1
  HDL Moving Average2/1 -> Signal Specification2/1
  Signal Specification1/1 -> Rate Transition1/1
  In2/1 -> HDL Moving Average1/1
  Rate Transition3/1 -> avgShort/1
  In1/1 -> HDL Moving Average/1
  Rate Transition/1 -> avgOpen/1
  Rate Transition1/1 -> avgUp/1
  Rate Transition2/1 -> avgDown/1
